simulink model "querySplit"  (R2024b)
settings: Solver=VariableStepAuto  StartTime=0.0  StopTime=10.0  RelTol=1e-3
settings Model: Creator=ryandavis  LastModifiedBy=ryandavis

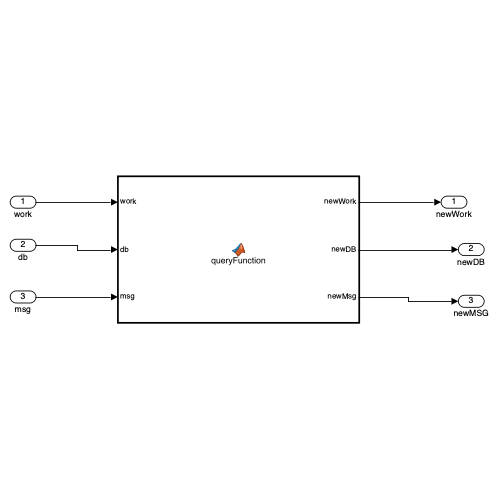
[thumbnail: Simulink's stored preview of the top-level diagram]
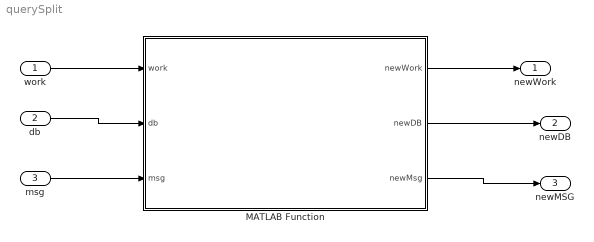
== system querySplit ==
  work : Inport
  db : Inport  Port=2
  msg : Inport  Port=3
  MATLAB Function : MATLAB Function  TreatAsAtomicUnit=on
  newWork : Outport
  newDB : Outport  Port=2
  newMSG : Outport  Port=3
  wires:
  work/1 -> MATLAB Function/1(work)
  db/1 -> MATLAB Function/2(db)
  msg/1 -> MATLAB Function/3(msg)
  MATLAB Function/1(newWork) -> newWork/1
  MATLAB Function/2(newDB) -> newDB/1
  MATLAB Function/3(newMsg) -> newMSG/1

== matlab function querySplit/MATLAB Function ==
  data: work input; newWork output; newDB output; db input; msg input; newMsg output
function [newWork, newDB, newMsg] = queryFunction(work, db, msg)
    
    newWork = work;
    newDB = db;
    newMsg = msg; 
end
